simulink model "BANSHEE"  (Simulink 8.1)
settings: Solver=ode1  StartTime=0.0  StopTime=inf  FixedStep=Ts  MaxStep=1e-3  RelTol=1e-3
model workspace (MAT data in the model file):
  op_snapshot1 : opcond.OperatingPoint (value not decoded)
PostLoadFcn:
  | BANSHEE_init;
InitFcn:
  | BANSHEE_init;
values from neighbouring files (symbols this model uses):
  Ts = 100E-6    (= 0.0001)    [BANSHEE_init.m]
undefined symbols (not defined in the file or in its folder): F1, F2, F3, fdesignblkfcn, Feeder1_lib, Feeder2_lib, Feeder3_lib, gcbh, generic_ethernet_cb, Left, relay_housing_lib, SM_UtilityService, SS_F1_RELAY_HOUSING, SS_F2_RELAY_HOUSING, SS_F3_RELAY_HOUSING, SS_Feeder1, SS_Feeder2, SS_Feeder3, type, utility_service_lib, V
libraries: breaker_lib x47, rtio_generic_modbus x43, relay_modbus_lib x42, cables_lib x41, transformer_lib x22, Load_lib x20, artemis x18, powerlib x18, rtio_opalrt_common x15, ssn_lib x15, rtlab x14, simulink x10
(part 1 of 5)
settings Model: ARTEMISmethode_block_infos=$$__separator__$$BANSHEE/ARTEMIS Guide$$__separator__$$  Creator=RE25624  LastModifiedBy=RE25624  BufferReuse=off
settings SolverCC: ZeroCrossAlgorithm=Adaptive
settings DataIOCC: ExternalInput=getinputstruct(op_snapshot1)  InitialState=getstatestruct(op_snapshot1)  LimitDataPoints=off  MaxDataPoints=90060  SignalLoggingSaveFormat=Dataset  SaveOutput=off  SignalLogging=off  DSMLogging=off  SaveTime=off  OutputSaveName=result
settings OptimizationCC: BlockReduction=off  OptimizeBlockIOStorage=off  BufferReuse=off  ExpressionFolding=off  LocalBlockOutputs=off
settings DebuggingCC: MaxConsecutiveZCsMsg=warning  IgnoredZcDiagnostic=none  SolverPrmCheckMsg=none  MultiTaskRateTransMsg=warning  FcnCallInpInsideContextMsg=EnableAllAsWarning  FrameProcessingCompatibilityMsg=error  ModelReferenceExtraNoncontSigs=warning  StrictBusMsg=None
settings ModelReferenceCC: UpdateModelReferenceTargets=IfOutOfDate
settings SFSimCC: SFSimEcho=off
settings GRTTargetCC: CodeReplacementLibrary=C89/C90 (ANSI)

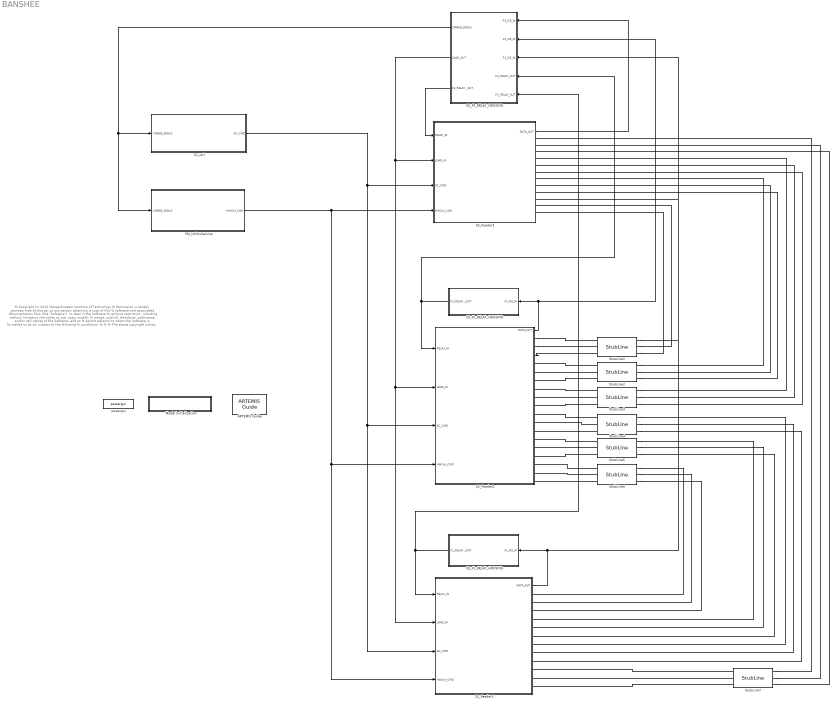
== system BANSHEE ==
  note: % Copyright (c) 2016 Massachusetts Institute of Technology
      | % Permission is hereby granted, free of charge, to any person obtaining a copy of this
      | % software and associated documentation files (the "Software"), to deal in the Software
      | % without restriction, including without limitation the rights to use, copy, modify,
      | % merge, publish, distribute, sublicense, and/or sell copies of the Software, and to
      | % permit persons to whom the Software is furnished to do so, subject to the following
      | % conditions:
      | %
      | %
      | % The above copyright notice and this permission notice shall be included in
      | % all copies or substantial portions of the Software.
      | %
      | % THE SOFTWARE IS PROVIDED "AS IS", WITHOUT WARRANTY OF ANY KIND, EXPRESS OR IMPLIED,
      | % INCLUDING BUT NOT LIMITED TO THE WARRANTIES OF MERCHANTABILITY, FITNESS FOR A
      | % PARTICULAR PURPOSE AND NONINFRINGEMENT. IN NO EVENT SHALL THE AUTHORS OR COPYRIGHT
      | % HOLDERS BE LIABLE FOR ANY CLAIM, DAMAGES OR OTHER LIABILITY, WHETHER IN AN ACTION
      | % OF CONTRACT, TORT OR OTHERWISE, ARISING FROM, OUT OF OR IN CONNECTION WITH THE
      | % SOFTWARE OR THE USE OR OTHER DEALINGS IN THE SOFTWARE.
      | %
      | %
      | %%
  ARTEMIS Guide : artemis/ARTEMIS/ARTEMIS Guide  Tag=FTSSmethode_opal_4hx0r99  Description=5.0_z1  lock=on  Ts=Ts  opt=art5  dyna=off  nb_perm=4  RT_fullcomp=off  ssn=on  ssn_itvc=off  ssn_ivic=off  ssn_ext=off  ssn_solver=Art5 with Backward Euler nodal interface  ssn_impulse=off  ssn_quasimpulse=off  ssn_impulse_loop=5  paraExtinctionThy=off  Thy_Impulse=on  dtc=Off  dtc_opt=normal  ao=on  simtype=off  ct_mac=off  lin_mov=off  lsp=[0.001 2]  spike_skip=Disabled  dtc_extra=1  dtc_sws=normal  dtc_pied=0.5  SPSRulesBlock=SPSRules  tre=on  ctmm=off  LF=off  dpl_type=ARTEMiS DPL  rlc_type=off  custom_type=off  para=on  ssn_ImpulseLoopBlockedStateUpdate=5  ssn_mov_iter_number=5  ssn_switch_iter_number=5
  Model Initialization : Subsystem  AncestorBlock=artemis/Tools /Misc/Model Initialization  mask(Model Functions){InitFcnX=BANSHEE_init;, prel=off, posl=on, inif=on, strf=off}
      mask prompts: InitFcnX "Initialisation"; prel "Preload Function"; posl "PostLoad Function"; inif "InitFcn"; strf "StartFcn"
      mask init:
      | currentBlock = gcb;
      | root = bdroot(currentBlock);
      | 
      | if ~strcmp(get_param(root,'BlockDiagramType'),'library')
      |     if prel==1
      |         set_param(root, 'PreLoadFcn', InitFcnX);
      |     else
      |         set_param(root, 'PreLoadFcn', '');
      |     end
      |     if inif==1
      |         set_param(root, 'InitFcn', InitFcnX);
      |     else
      |         set_param(root, 'InitFcn', '');
      |     end
      |     if strf==1
      |         set_param(root, 'StartFcn', InitFcnX);
      |     else
      |         set_param(root, 'StartFcn', '');
      |     end
      |     if posl==1
      |         set_param(root, 'PostLoadFcn', InitFcnX);
      |     else
      |         set_param(root, 'PostLoadFcn', '');
      |     end
      | end
      | 
      | pos = get_param(currentBlock, 'Position');
      | width = pos(3) - pos(1); height = pos(4) - pos(2);
      | txt = [ upper(root) '\n' '- InitFcn. . . . . '  get_param(root, 'InitFcn') ];
      settings: CopyFcn=set_param(gcb,'LinkStatus','inactive')
      mask Display: text(5, height*0.5, txt, 'horizontalAlignment', 'left', 'verticalAlignment', 'middle') ;
  SC_ctrl : Subsystem
  SM_UtilityService : Subsystem  AncestorBlock=utility_service_lib/SM_UtilityService
  SS_F1_RELAY_HOUSING : Subsystem  AncestorBlock=relay_housing_lib/SS_F1_RELAY_HOUSING
  SS_F2_RELAY_HOUSING : Subsystem  AncestorBlock=relay_housing_lib/SS_F2_RELAY_HOUSING
  SS_F3_RELAY_HOUSING : Subsystem  AncestorBlock=relay_housing_lib/SS_F3_RELAY_HOUSING
  SS_Feeder1 : Subsystem  AncestorBlock=Feeder1_lib/SS_Feeder1
  SS_Feeder2 : Subsystem  AncestorBlock=Feeder2_lib/SS_Feeder2
  SS_Feeder3 : Subsystem  AncestorBlock=Feeder3_lib/SS_Feeder3
  StubLine1 : artemis/ARTEMIS/StubLine  Phases=3  pu=off  L=1500 * 9.43453e-08 / 2  Lpu=0.08  R=1500 * 2.28409e-5 / 2  Rpu=0.002  S_base=450e6/3  V_base=230e3/sqrt(3)  F_base=60  Ts=Ts
  StubLine2 : artemis/ARTEMIS/StubLine  Phases=3  pu=off  L=1500 * 9.43453e-08 / 2  Lpu=0.08  R=1500 * 2.28409e-5 / 2  Rpu=0.002  S_base=450e6/3  V_base=230e3/sqrt(3)  F_base=60  Ts=Ts
  StubLine3 : artemis/ARTEMIS/StubLine  Phases=3  pu=off  L=1500 * 9.43453e-08 / 2  Lpu=0.08  R=1500 * 2.28409e-5 / 2  Rpu=0.002  S_base=450e6/3  V_base=230e3/sqrt(3)  F_base=60  Ts=Ts
  StubLine4 : artemis/ARTEMIS/StubLine  Phases=3  pu=off  L=1000 * 9.43453e-08 / 2  Lpu=0.08  R=1000 * 2.28409e-5 / 2  Rpu=0.002  S_base=450e6/3  V_base=230e3/sqrt(3)  F_base=60  Ts=Ts
  StubLine5 : artemis/ARTEMIS/StubLine  Phases=3  pu=off  L=2000 * 9.43453e-08 / 2  Lpu=0.08  R=2000 * 2.28409e-5 / 2  Rpu=0.002  S_base=450e6/3  V_base=230e3/sqrt(3)  F_base=60  Ts=Ts
  StubLine6 : artemis/ARTEMIS/StubLine  Phases=3  pu=off  L=3000 * 9.43453e-08 / 1  Lpu=0.08  R=3000 * 2.28409e-5 / 1  Rpu=0.002  S_base=450e6/3  V_base=230e3/sqrt(3)  F_base=60  Ts=Ts
  StubLine7 : artemis/ARTEMIS/StubLine  Phases=3  pu=off  L=2000 * 9.43453e-08 / 2  Lpu=0.08  R=2000 * 2.28409e-5 / 2  Rpu=0.002  S_base=450e6/3  V_base=230e3/sqrt(3)  F_base=60  Ts=Ts
  powergui : powerlib/powergui  Priority=2  SimulationMode=Discrete  SolverType=Tustin  SampleTime=Ts  frequency=60  SPID=off  DisableSnubberDevices=off  DisableRonSwitches=off  DisableVfSwitches=off  SwTol=0  Interpol=off  DisplayEquations=off  frequencyindice=0  Pbase=100e6  ErrMax=1e-4  Iterations=50  UnitsV=kV  UnitsW=MW  FunctionMessages=off  echomessages=off  HookPort=off  EnableUseOfTLC=off  x0status=blocks  RestoreLinks=warning  ResistiveCurrentMeasurement=off  Frange=logspace(0,3,50)  Ylog=off  Xlog=off  ShowGrid=off  save=off  variable=ZData  structure=0  ZoomFFT=on  StartTime=0.0  cycles=2  DisplayStyle=off  fundamental=60  FreqAxis=off  MaxFrequency=1000  frequencyindicesteady=1  RmsSteady=1  display=off  Ts=0  methode=off
  wires:
  SS_Feeder3/1(DATA_OUT) -> SS_F3_RELAY_HOUSING/1(F3_MS_IN)
  SS_F3_RELAY_HOUSING/3(F3_RELAY _OUT) -> SS_Feeder3/1(RELAY_IN)
  SS_F1_RELAY_HOUSING/1(F1_RELAY _OUT) -> SS_Feeder1/1(RELAY_IN), SS_F3_RELAY_HOUSING/5(F1_RELAY_OUT)
  SS_F2_RELAY_HOUSING/1(F2_RELAY _OUT) -> SS_F3_RELAY_HOUSING/4(F2_RELAY_OUT), SS_Feeder2/1(RELAY_IN)
  SS_Feeder1/1(DATA_OUT) -> SS_F3_RELAY_HOUSING/3(F1_MS_IN), SS_F1_RELAY_HOUSING/1(F1_MS_IN)
  SS_Feeder2/1(DATA_OUT) -> SS_F3_RELAY_HOUSING/2(F2_MS_IN), SS_F2_RELAY_HOUSING/1(F2_MS_IN)
  SC_ctrl/1(SC_CMD) -> SS_Feeder1/3(SC_CMD), SS_Feeder2/3(SC_CMD), SS_Feeder3/3(SC_CMD)
  SS_F3_RELAY_HOUSING/2(LOAD_OUT) -> SS_Feeder3/2(LOAD_IN), SS_Feeder1/2(LOAD_IN), SS_Feeder2/2(LOAD_IN)
  SM_UtilityService/1(HWCtrl_CMD) -> SS_Feeder1/4(HWCtrl_CMD), SS_Feeder2/4(HWCtrl_CMD), SS_Feeder3/4(HWCtrl_CMD)
  SS_F3_RELAY_HOUSING/1(CMBNE_SGNLS) -> SM_UtilityService/1(CMBNE_SGNLS), SC_ctrl/1(CMBNE_SGNLS)
  connections:
  SS_Feeder2/RConn2 -- StubLine1/LConn2
  SS_Feeder2/RConn1 -- StubLine1/LConn1
  SS_Feeder2/RConn3 -- StubLine1/LConn3
  StubLine2/LConn2 -- SS_Feeder2/RConn5
  StubLine2/LConn3 -- SS_Feeder2/RConn6
  StubLine2/LConn1 -- SS_Feeder2/RConn4
  StubLine3/LConn2 -- SS_Feeder2/RConn8
  StubLine3/LConn1 -- SS_Feeder2/RConn7
  StubLine3/LConn3 -- SS_Feeder2/RConn9
  StubLine4/LConn3 -- SS_Feeder2/RConn12
  StubLine4/LConn2 -- SS_Feeder2/RConn11
  StubLine4/LConn1 -- SS_Feeder2/RConn10
  StubLine7/LConn3 -- SS_Feeder1/RConn12
  StubLine7/LConn2 -- SS_Feeder1/RConn11
  StubLine7/LConn1 -- SS_Feeder1/RConn10
  StubLine5/LConn2 -- SS_Feeder2/RConn14
  StubLine5/LConn1 -- SS_Feeder2/RConn13
  StubLine5/LConn3 -- SS_Feeder2/RConn15
  StubLine6/LConn3 -- SS_Feeder2/RConn18
  StubLine6/LConn2 -- SS_Feeder2/RConn17
  StubLine6/LConn1 -- SS_Feeder2/RConn16
  StubLine6/RConn1 -- SS_Feeder1/RConn1
  StubLine6/RConn2 -- SS_Feeder1/RConn2
  StubLine6/RConn3 -- SS_Feeder1/RConn3
  StubLine5/RConn1 -- SS_Feeder1/RConn4
  StubLine5/RConn2 -- SS_Feeder1/RConn5
  StubLine5/RConn3 -- SS_Feeder1/RConn6
  StubLine4/RConn1 -- SS_Feeder1/RConn7
  StubLine4/RConn2 -- SS_Feeder1/RConn8
  StubLine4/RConn3 -- SS_Feeder1/RConn9
  StubLine3/RConn3 -- SS_Feeder3/RConn6
  StubLine3/RConn2 -- SS_Feeder3/RConn5
  StubLine3/RConn1 -- SS_Feeder3/RConn4
  StubLine2/RConn3 -- SS_Feeder3/RConn9
  StubLine2/RConn2 -- SS_Feeder3/RConn8
  StubLine2/RConn1 -- SS_Feeder3/RConn7
  StubLine1/RConn3 -- SS_Feeder3/RConn12
  StubLine1/RConn2 -- SS_Feeder3/RConn11
  StubLine1/RConn1 -- SS_Feeder3/RConn10
  StubLine7/RConn1 -- SS_Feeder3/RConn1
  StubLine7/RConn2 -- SS_Feeder3/RConn2
  StubLine7/RConn3 -- SS_Feeder3/RConn3

== system BANSHEE/Model Initialization ==

== system BANSHEE/SC_ctrl ==
  note: % Copyright (c) 2016 Massachusetts Institute of Technology
      | % Permission is hereby granted, free of charge, to any person obtaining a copy of this
      | % software and associated documentation files (the "Software"), to deal in the Software
      | % without restriction, including without limitation the rights to use, copy, modify,
      | % merge, publish, distribute, sublicense, and/or sell copies of the Software, and to
      | % permit persons to whom the Software is furnished to do so, subject to the following
      | % conditions:
      | %
      | %
      | % The above copyright notice and this permission notice shall be included in
      | % all copies or substantial portions of the Software.
      | %
      | % THE SOFTWARE IS PROVIDED "AS IS", WITHOUT WARRANTY OF ANY KIND, EXPRESS OR IMPLIED,
      | % INCLUDING BUT NOT LIMITED TO THE WARRANTIES OF MERCHANTABILITY, FITNESS FOR A
      | % PARTICULAR PURPOSE AND NONINFRINGEMENT. IN NO EVENT SHALL THE AUTHORS OR COPYRIGHT
      | % HOLDERS BE LIABLE FOR ANY CLAIM, DAMAGES OR OTHER LIABILITY, WHETHER IN AN ACTION
      | % OF CONTRACT, TORT OR OTHERWISE, ARISING FROM, OUT OF OR IN CONNECTION WITH THE
      | % SOFTWARE OR THE USE OR OTHER DEALINGS IN THE SOFTWARE.
      | %
      | %
      | %%
  note: The 'Overruns' value should remain at 0.
      | The 'Ttotal' value should be equal to the
      | model Fixed-Step size.
  CMBNE_SGNLS : Inport
  Bus Creator : BusCreator  Inputs=2
  Bus Creator1 : BusCreator  Inputs=3
  Bus Selector : BusSelector  OutputSignals=F1_RELAY_OUT,F2_RELAY_OUT,F3_RELAY_OUT
  F1 : Subsystem
  F1 1: connect motor 0: disconnect motor1 : Constant  Value=0
  F2 : Subsystem
  F3 : Subsystem
  F3 1: connect motor 0: disconnect motor : Constant  Value=0
  OpComm : rtlab/OpComm  nbport=1  groupe_acq=1  subsys_rate=0  st=0  Synchronization=on  Interpolation=on  Threshold=1.0  Missed_Data=off  Sim_Time=off  Samples=off  dynSigOut=off  from_console=0  warning_done=off  writeOpCommFile=off  Offset=off
  Woodward : Subsystem
  opElectricFaultSelector : artemis/Tools /POW faults/opElectricFaultSelector  phase_a=on  phase_b=on  phase_c=on  gnd_fault=on  Tacq=1  Tst=[0.1 0 10]  enable_POW=off  angle_POW=[15 0 10]  Tdr="[0.5 0  10]"  fault_location_menu=No fault  T_init=2
  SC_CMD : Outport
  wires:
  CMBNE_SGNLS/1 -> OpComm/1
  opElectricFaultSelector/1 -> [fault_cmd]
  Bus Creator1/1 -> SC_CMD/1
  [IO_ctrl] -> Bus Creator1/3  "IO ctrl"
  Woodward/1(IOctrl) -> [IO_ctrl]
  [fault_cmd] -> Bus Creator1/1  "fault_cmd"
  OpComm/1 -> Bus Selector/1
  Bus Creator/1 -> Bus Creator1/2  "motor_ONOFF"
  F3 1: connect motor 0: disconnect motor/1 -> Bus Creator/1  "F3_motor_ONOFF"
  F1 1: connect motor 0: disconnect motor1/1 -> Bus Creator/2  "F1_motor_ONOFF"
  Bus Selector/1 -> F1/1(F1)  "<F1_RELAY_OUT>"
  Bus Selector/3 -> F3/1(F3)  "<F3_RELAY_OUT>"
  Bus Selector/2 -> F2/1(F2)  "<F2_RELAY_OUT>"

== system BANSHEE/SM_UtilityService ==
  note: % Copyright (c) 2016 Massachusetts Institute of Technology
      | % Permission is hereby granted, free of charge, to any person obtaining a copy of this
      | % software and associated documentation files (the "Software"), to deal in the Software
      | % without restriction, including without limitation the rights to use, copy, modify,
      | % merge, publish, distribute, sublicense, and/or sell copies of the Software, and to
      | % permit persons to whom the Software is furnished to do so, subject to the following
      | % conditions:
      | %
      | %
      | % The above copyright notice and this permission notice shall be included in
      | % all copies or substantial portions of the Software.
      | %
      | % THE SOFTWARE IS PROVIDED "AS IS", WITHOUT WARRANTY OF ANY KIND, EXPRESS OR IMPLIED,
      | % INCLUDING BUT NOT LIMITED TO THE WARRANTIES OF MERCHANTABILITY, FITNESS FOR A
      | % PARTICULAR PURPOSE AND NONINFRINGEMENT. IN NO EVENT SHALL THE AUTHORS OR COPYRIGHT
      | % HOLDERS BE LIABLE FOR ANY CLAIM, DAMAGES OR OTHER LIABILITY, WHETHER IN AN ACTION
      | % OF CONTRACT, TORT OR OTHERWISE, ARISING FROM, OUT OF OR IN CONNECTION WITH THE
      | % SOFTWARE OR THE USE OR OTHER DEALINGS IN THE SOFTWARE.
      | %
      | %
      | %%
  CMBNE_SGNLS : Inport
  2X MCB - Genset_signal_scaling - 3.5MVA : EasyGen3500_GensetSignalScaling_lib/2X MCB - Genset_signal_scaling - 3.5MVA  Vpk_mcb=11268  watt_mcb=3150000  Vpk_gcb=11268  watt_gcb=3150000  rated_rpm=1800  wm_noise_bias=0.02
  Bus Creator4 : BusCreator  Inputs=3
  Bus Selector1 : BusSelector  OutputSignals="F1_MS_IN.DIESEL_DATA.DIESEL_GCB.cb_ms,F1_MS_IN.CB_DATA.F1_PCC,F1_MS_IN.DIESEL_DATA.Gen2_meas.w.w.Rotor speed  wm (pu)"
  Bus Selector2 : BusSelector  OutputSignals=F1_MS_IN.CB_DATA.F1_PCC,F2_MS_IN.CB_DATA.F2_PCC,F3_MS_IN.CB_DATA.F3_PCC
  Bus Selector4 : BusSelector  OutputSignals="F3_MS_IN.NG_CHP_DATA.NG_CHP_GCB.cb_ms,F3_MS_IN.CB_DATA.F3_PCC,F3_MS_IN.NG_CHP_DATA.Gen1_meas.w.w.Rotor speed  wm (pu),F3_MS_IN.CB_DATA.F3_CB_3"
  Genset_signal_scaling - 4MVA : EasyGen3500_GensetSignalScaling_lib/Genset_signal_scaling - 4MVA  Vpk_mcb=11268  watt_mcb=3600000  Vpk_gcb=11268  watt_gcb=3600000  rated_rpm=1800  wm_noise_bias=0.02
  HWCtrl_IOs : Subsystem
  Memory1 : Memory
  OpComm2 : rtlab/OpComm  nbport=1  groupe_acq=1  subsys_rate=0  st=0  Synchronization=on  Interpolation=on  Threshold=1.0  Missed_Data=off  Sim_Time=off  Samples=off  dynSigOut=off  from_console=0  warning_done=off  writeOpCommFile=off  Offset=off
  SEL751 - SignalScaling : Subsystem  mask(SEL751 - SignalScaling){ct_ratio=1/1250, pt_ratio=1/1800}
      mask prompts: ct_ratio "CT Ratio"; pt_ratio "PT Ratio"
      mask help: CT and PT ratios should match the settings in the corresponding SEL751
  HWCtrl_CMD : Outport
  wires:
  Memory1/1 -> HWCtrl_CMD/1
  2X MCB - Genset_signal_scaling - 3.5MVA/1 -> Bus Creator4/1  "NGCHP_ScaledSignals"
  Genset_signal_scaling - 4MVA/1 -> Bus Creator4/2  "Diesel_ScaledSignals"
  [CMBNE_SGNLS] -> Bus Selector4/1, Bus Selector2/1, Bus Selector1/1  "MCB"
  Bus Selector4/3 -> 2X MCB - Genset_signal_scaling - 3.5MVA/3  "<Rotor speed  wm (pu)>"
  Bus Selector4/2 -> 2X MCB - Genset_signal_scaling - 3.5MVA/2  "<F3_PCC>"
  Bus Selector4/1 -> 2X MCB - Genset_signal_scaling - 3.5MVA/1  "<cb_ms>"
  Bus Creator4/1 -> HWCtrl_IOs/1(ScaledSignals)
  HWCtrl_IOs/1(WoodwardBias) -> Memory1/1
  Bus Selector1/3 -> Genset_signal_scaling - 4MVA/3  "<Rotor speed  wm (pu)>"
  Bus Selector1/2 -> Genset_signal_scaling - 4MVA/2  "<F1_PCC>"
  Bus Selector1/1 -> Genset_signal_scaling - 4MVA/1  "<cb_ms>"
  CMBNE_SGNLS/1 -> OpComm2/1
  OpComm2/1 -> [CMBNE_SGNLS]
  SEL751 - SignalScaling/1(ScaledSignals) -> Bus Creator4/3  "SEL751_ScaledSignals"
  Bus Selector2/2 -> SEL751 - SignalScaling/2(Relay_F2)  "<F2_PCC>"
  Bus Selector2/1 -> SEL751 - SignalScaling/1(Relay_F1)  "<F1_PCC>"
  Bus Selector2/3 -> SEL751 - SignalScaling/3(Relay_F3)  "<F3_PCC>"
  Bus Selector4/4 -> 2X MCB - Genset_signal_scaling - 3.5MVA/4  "<F3_CB_3>"

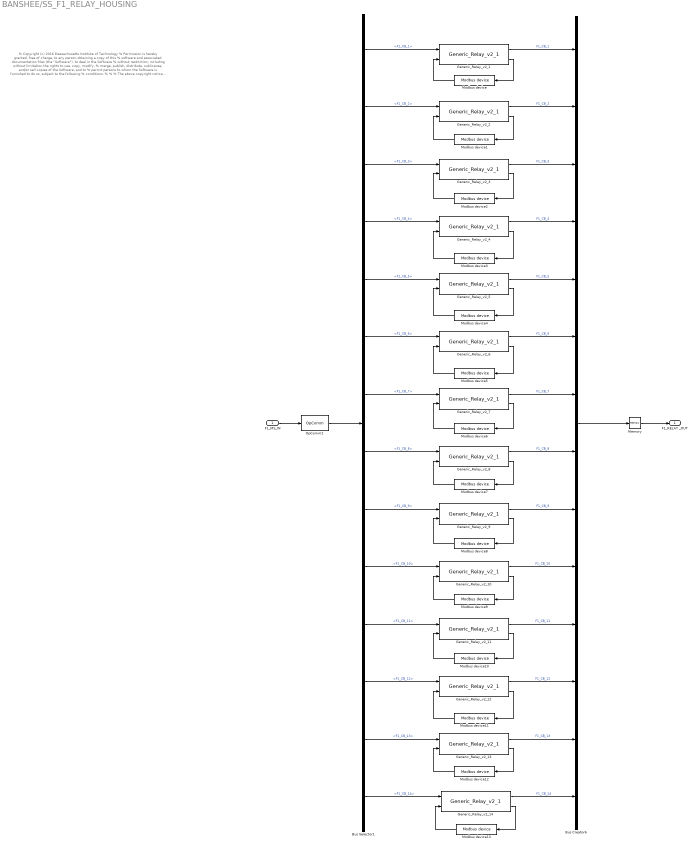
== system BANSHEE/SS_F1_RELAY_HOUSING ==
  note: % Copyright (c) 2016 Massachusetts Institute of Technology
      | % Permission is hereby granted, free of charge, to any person obtaining a copy of this
      | % software and associated documentation files (the "Software"), to deal in the Software
      | % without restriction, including without limitation the rights to use, copy, modify,
      | % merge, publish, distribute, sublicense, and/or sell copies of the Software, and to
      | % permit persons to whom the Software is furnished to do so, subject to the following
      | % conditions:
      | %
      | %
      | % The above copyright notice and this permission notice shall be included in
      | % all copies or substantial portions of the Software.
      | %
      | % THE SOFTWARE IS PROVIDED "AS IS", WITHOUT WARRANTY OF ANY KIND, EXPRESS OR IMPLIED,
      | % INCLUDING BUT NOT LIMITED TO THE WARRANTIES OF MERCHANTABILITY, FITNESS FOR A
      | % PARTICULAR PURPOSE AND NONINFRINGEMENT. IN NO EVENT SHALL THE AUTHORS OR COPYRIGHT
      | % HOLDERS BE LIABLE FOR ANY CLAIM, DAMAGES OR OTHER LIABILITY, WHETHER IN AN ACTION
      | % OF CONTRACT, TORT OR OTHERWISE, ARISING FROM, OUT OF OR IN CONNECTION WITH THE
      | % SOFTWARE OR THE USE OR OTHER DEALINGS IN THE SOFTWARE.
      | %
      | %
      | %%
  F1_MS_IN : Inport
  Bus Creator6 : BusCreator  Inputs=14
  Bus Selector1 : BusSelector  OutputSignals=CB_DATA.F1_CB_1,CB_DATA.F1_CB_2,CB_DATA.F1_CB_3,CB_DATA.F1_CB_4,CB_DATA.F1_CB_5,CB_DATA.F1_CB_6,CB_DATA.F1_CB_7,CB_DATA.F1_CB_8,CB_DATA.F1_CB_9,CB_DATA.F1_CB_10,CB_DATA.F1_CB_11,CB_DATA.F1_CB_12,CB_DATA.F1_CB_13,CB_DATA.F1_CB_14
  Generic_Relay_v2_1 : relay_modbus_lib/Generic_Relay_v2_1  Ts=Ts  relay_settings=[F1(1,:)]
  Generic_Relay_v2_10 : relay_modbus_lib/Generic_Relay_v2_1  Ts=Ts  relay_settings=[F1(10,:)]
  Generic_Relay_v2_11 : relay_modbus_lib/Generic_Relay_v2_1  Ts=Ts  relay_settings=[F1(11,:)]
  Generic_Relay_v2_12 : relay_modbus_lib/Generic_Relay_v2_1  Ts=Ts  relay_settings=[F1(12,:)]
  Generic_Relay_v2_13 : relay_modbus_lib/Generic_Relay_v2_1  Ts=Ts  relay_settings=[F1(13,:)]
  Generic_Relay_v2_14 : relay_modbus_lib/Generic_Relay_v2_1  Ts=Ts  relay_settings=[F1(14,:)]
  Generic_Relay_v2_2 : relay_modbus_lib/Generic_Relay_v2_1  Ts=Ts  relay_settings=[F1(2,:)]
  Generic_Relay_v2_3 : relay_modbus_lib/Generic_Relay_v2_1  Ts=Ts  relay_settings=[F1(3,:)]
  Generic_Relay_v2_4 : relay_modbus_lib/Generic_Relay_v2_1  Ts=Ts  relay_settings=[F1(4,:)]
  Generic_Relay_v2_5 : relay_modbus_lib/Generic_Relay_v2_1  Ts=Ts  relay_settings=[F1(5,:)]
  Generic_Relay_v2_6 : relay_modbus_lib/Generic_Relay_v2_1  Ts=Ts  relay_settings=[F1(6,:)]
  Generic_Relay_v2_7 : relay_modbus_lib/Generic_Relay_v2_1  Ts=Ts  relay_settings=[F1(7,:)]
  Generic_Relay_v2_8 : relay_modbus_lib/Generic_Relay_v2_1  Ts=Ts  relay_settings=[F1(8,:)]
  Generic_Relay_v2_9 : relay_modbus_lib/Generic_Relay_v2_1  Ts=Ts  relay_settings=[F1(9,:)]
  Memory : Memory
  Modbus device : rtio_generic_modbus/Modbus device  conf_name=F1_relay_cfg1.opal  conf_name_mask=F1_relay_cfg1.xls  sample_time=Ts
  Modbus device1 : rtio_generic_modbus/Modbus device  conf_name=F1_relay_cfg2.opal  conf_name_mask=F1_relay_cfg2.xls  sample_time=Ts
  Modbus device10 : rtio_generic_modbus/Modbus device  conf_name=F1_relay_cfg11.opal  conf_name_mask=F1_relay_cfg11.xls  sample_time=Ts
  Modbus device11 : rtio_generic_modbus/Modbus device  conf_name=F1_relay_cfg12.opal  conf_name_mask=F1_relay_cfg12.xls  sample_time=Ts
  Modbus device12 : rtio_generic_modbus/Modbus device  conf_name=F1_relay_cfg13.opal  conf_name_mask=F1_relay_cfg13.xls  sample_time=Ts
  Modbus device13 : rtio_generic_modbus/Modbus device  conf_name=F1_relay_cfg14.opal  conf_name_mask=F1_relay_cfg14.xls  sample_time=Ts
  Modbus device2 : rtio_generic_modbus/Modbus device  conf_name=F1_relay_cfg3.opal  conf_name_mask=F1_relay_cfg3.xls  sample_time=Ts
  Modbus device3 : rtio_generic_modbus/Modbus device  conf_name=F1_relay_cfg4.opal  conf_name_mask=F1_relay_cfg4.xls  sample_time=Ts
  Modbus device4 : rtio_generic_modbus/Modbus device  conf_name=F1_relay_cfg5.opal  conf_name_mask=F1_relay_cfg5.xls  sample_time=Ts
  Modbus device5 : rtio_generic_modbus/Modbus device  conf_name=F1_relay_cfg6.opal  conf_name_mask=F1_relay_cfg6.xls  sample_time=Ts
  Modbus device6 : rtio_generic_modbus/Modbus device  conf_name=F1_relay_cfg7.opal  conf_name_mask=F1_relay_cfg7.xls  sample_time=Ts
  Modbus device7 : rtio_generic_modbus/Modbus device  conf_name=F1_relay_cfg8.opal  conf_name_mask=F1_relay_cfg8.xls  sample_time=Ts
  Modbus device8 : rtio_generic_modbus/Modbus device  conf_name=F1_relay_cfg9.opal  conf_name_mask=F1_relay_cfg9.xls  sample_time=Ts
  Modbus device9 : rtio_generic_modbus/Modbus device  conf_name=F1_relay_cfg10.opal  conf_name_mask=F1_relay_cfg10.xls  sample_time=Ts
  OpComm2 : rtlab/OpComm  nbport=1  groupe_acq=1  subsys_rate=0  st=0  Synchronization=on  Interpolation=on  Threshold=1.0  Missed_Data=off  Sim_Time=off  Samples=off  dynSigOut=off  from_console=0  warning_done=off  writeOpCommFile=off  Offset=off
  F1_RELAY _OUT : Outport
  wires:
  OpComm2/1 -> Bus Selector1/1
  Modbus device12/1 -> Generic_Relay_v2_13/2
  Generic_Relay_v2_13/2 -> Modbus device12/1
  Modbus device11/1 -> Generic_Relay_v2_12/2
  Generic_Relay_v2_12/2 -> Modbus device11/1
  Modbus device10/1 -> Generic_Relay_v2_11/2
  Generic_Relay_v2_11/2 -> Modbus device10/1
  Modbus device9/1 -> Generic_Relay_v2_10/2
  Generic_Relay_v2_10/2 -> Modbus device9/1
  Modbus device8/1 -> Generic_Relay_v2_9/2
  Generic_Relay_v2_9/2 -> Modbus device8/1
  Modbus device7/1 -> Generic_Relay_v2_8/2
  Generic_Relay_v2_8/2 -> Modbus device7/1
  Modbus device6/1 -> Generic_Relay_v2_7/2
  Generic_Relay_v2_7/2 -> Modbus device6/1
  Modbus device5/1 -> Generic_Relay_v2_6/2
  Generic_Relay_v2_6/2 -> Modbus device5/1
  Modbus device4/1 -> Generic_Relay_v2_5/2
  Generic_Relay_v2_5/2 -> Modbus device4/1
  Modbus device3/1 -> Generic_Relay_v2_4/2
  Generic_Relay_v2_4/2 -> Modbus device3/1
  Modbus device2/1 -> Generic_Relay_v2_3/2
  Generic_Relay_v2_3/2 -> Modbus device2/1
  Generic_Relay_v2_2/2 -> Modbus device1/1
  Modbus device1/1 -> Generic_Relay_v2_2/2
  Generic_Relay_v2_1/2 -> Modbus device/1
  Modbus device/1 -> Generic_Relay_v2_1/2
  F1_MS_IN/1 -> OpComm2/1
  Bus Selector1/1 -> Generic_Relay_v2_1/1  "<F1_CB_1>"
  Generic_Relay_v2_1/1 -> Bus Creator6/1  "F1_CB_1"
  Bus Creator6/1 -> Memory/1
  Bus Selector1/2 -> Generic_Relay_v2_2/1  "<F1_CB_2>"
  Generic_Relay_v2_2/1 -> Bus Creator6/2  "F1_CB_2"
  Bus Selector1/3 -> Generic_Relay_v2_3/1  "<F1_CB_3>"
  Bus Selector1/4 -> Generic_Relay_v2_4/1  "<F1_CB_4>"
  Bus Selector1/5 -> Generic_Relay_v2_5/1  "<F1_CB_5>"
  Bus Selector1/6 -> Generic_Relay_v2_6/1  "<F1_CB_6>"
  Bus Selector1/7 -> Generic_Relay_v2_7/1  "<F1_CB_7>"
  Bus Selector1/8 -> Generic_Relay_v2_8/1  "<F1_CB_8>"
  Bus Selector1/9 -> Generic_Relay_v2_9/1  "<F1_CB_9>"
  Bus Selector1/10 -> Generic_Relay_v2_10/1  "<F1_CB_10>"
  Bus Selector1/11 -> Generic_Relay_v2_11/1  "<F1_CB_11>"
  Bus Selector1/12 -> Generic_Relay_v2_12/1  "<F1_CB_12>"
  Bus Selector1/13 -> Generic_Relay_v2_13/1  "<F1_CB_13>"
  Generic_Relay_v2_13/1 -> Bus Creator6/13  "F1_CB_13"
  Generic_Relay_v2_12/1 -> Bus Creator6/12  "F1_CB_12"
  Generic_Relay_v2_11/1 -> Bus Creator6/11  "F1_CB_11"
  Generic_Relay_v2_10/1 -> Bus Creator6/10  "F1_CB_10"
  Generic_Relay_v2_9/1 -> Bus Creator6/9  "F1_CB_9"
  Generic_Relay_v2_8/1 -> Bus Creator6/8  "F1_CB_8"
  Generic_Relay_v2_7/1 -> Bus Creator6/7  "F1_CB_7"
  Generic_Relay_v2_6/1 -> Bus Creator6/6  "F1_CB_6"
  Generic_Relay_v2_5/1 -> Bus Creator6/5  "F1_CB_5"
  Generic_Relay_v2_4/1 -> Bus Creator6/4  "F1_CB_4"
  Generic_Relay_v2_3/1 -> Bus Creator6/3  "F1_CB_3"
  Modbus device13/1 -> Generic_Relay_v2_14/2
  Generic_Relay_v2_14/2 -> Modbus device13/1
  Generic_Relay_v2_14/1 -> Bus Creator6/14  "F1_CB_14"
  Bus Selector1/14 -> Generic_Relay_v2_14/1  "<F1_CB_14>"
  Memory/1 -> F1_RELAY _OUT/1

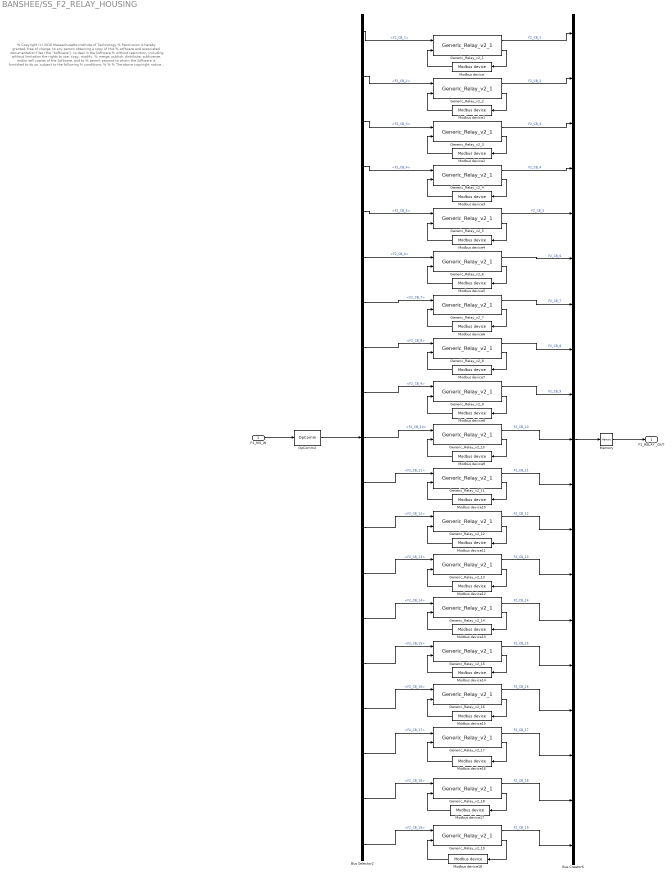
== system BANSHEE/SS_F2_RELAY_HOUSING ==
  note: % Copyright (c) 2016 Massachusetts Institute of Technology
      | % Permission is hereby granted, free of charge, to any person obtaining a copy of this
      | % software and associated documentation files (the "Software"), to deal in the Software
      | % without restriction, including without limitation the rights to use, copy, modify,
      | % merge, publish, distribute, sublicense, and/or sell copies of the Software, and to
      | % permit persons to whom the Software is furnished to do so, subject to the following
      | % conditions:
      | %
      | %
      | % The above copyright notice and this permission notice shall be included in
      | % all copies or substantial portions of the Software.
      | %
      | % THE SOFTWARE IS PROVIDED "AS IS", WITHOUT WARRANTY OF ANY KIND, EXPRESS OR IMPLIED,
      | % INCLUDING BUT NOT LIMITED TO THE WARRANTIES OF MERCHANTABILITY, FITNESS FOR A
      | % PARTICULAR PURPOSE AND NONINFRINGEMENT. IN NO EVENT SHALL THE AUTHORS OR COPYRIGHT
      | % HOLDERS BE LIABLE FOR ANY CLAIM, DAMAGES OR OTHER LIABILITY, WHETHER IN AN ACTION
      | % OF CONTRACT, TORT OR OTHERWISE, ARISING FROM, OUT OF OR IN CONNECTION WITH THE
      | % SOFTWARE OR THE USE OR OTHER DEALINGS IN THE SOFTWARE.
      | %
      | %
      | %%
  F2_MS_IN : Inport
  Bus Creator6 : BusCreator  Inputs=19
  Bus Selector2 : BusSelector  OutputSignals=CB_DATA.F2_CB_1,CB_DATA.F2_CB_2,CB_DATA.F2_CB_3,CB_DATA.F2_CB_4,CB_DATA.F2_CB_5,CB_DATA.F2_CB_6,CB_DATA.F2_CB_7,CB_DATA.F2_CB_8,CB_DATA.F2_CB_9,CB_DATA.F2_CB_10,CB_DATA.F2_CB_11,CB_DATA.F2_CB_12,CB_DATA.F2_CB_13,CB_DATA.F2_CB_14,CB_DATA.F2_CB_15,CB_DATA.F2_CB_16,CB_DATA.F2_CB_17,CB_DATA.F2_CB_18,CB_DATA.F2_CB_19
  Generic_Relay_v2_1 : relay_modbus_lib/Generic_Relay_v2_1  Ts=Ts  relay_settings=[F2(1,:)]
  Generic_Relay_v2_10 : relay_modbus_lib/Generic_Relay_v2_1  Ts=Ts  relay_settings=[F2(10,:)]
  Generic_Relay_v2_11 : relay_modbus_lib/Generic_Relay_v2_1  Ts=Ts  relay_settings=[F2(11,:)]
  Generic_Relay_v2_12 : relay_modbus_lib/Generic_Relay_v2_1  Ts=Ts  relay_settings=[F2(12,:)]
  Generic_Relay_v2_13 : relay_modbus_lib/Generic_Relay_v2_1  Ts=Ts  relay_settings=[F2(13,:)]
  Generic_Relay_v2_14 : relay_modbus_lib/Generic_Relay_v2_1  Ts=Ts  relay_settings=[F2(14,:)]
  Generic_Relay_v2_15 : relay_modbus_lib/Generic_Relay_v2_1  Ts=Ts  relay_settings=[F2(15,:)]
  Generic_Relay_v2_16 : relay_modbus_lib/Generic_Relay_v2_1  Ts=Ts  relay_settings=[F2(16,:)]
  Generic_Relay_v2_17 : relay_modbus_lib/Generic_Relay_v2_1  Ts=Ts  relay_settings=[F2(17,:)]
  Generic_Relay_v2_18 : relay_modbus_lib/Generic_Relay_v2_1  Ts=Ts  relay_settings=[F2(18,:)]
  Generic_Relay_v2_19 : relay_modbus_lib/Generic_Relay_v2_1  Ts=Ts  relay_settings=[F2(19,:)]
  Generic_Relay_v2_2 : relay_modbus_lib/Generic_Relay_v2_1  Ts=Ts  relay_settings=[F2(2,:)]
  Generic_Relay_v2_3 : relay_modbus_lib/Generic_Relay_v2_1  Ts=Ts  relay_settings=[F2(3,:)]
  Generic_Relay_v2_4 : relay_modbus_lib/Generic_Relay_v2_1  Ts=Ts  relay_settings=[F2(4,:)]
  Generic_Relay_v2_5 : relay_modbus_lib/Generic_Relay_v2_1  Ts=Ts  relay_settings=[F2(5,:)]
  Generic_Relay_v2_6 : relay_modbus_lib/Generic_Relay_v2_1  Ts=Ts  relay_settings=[F2(6,:)]
  Generic_Relay_v2_7 : relay_modbus_lib/Generic_Relay_v2_1  Ts=Ts  relay_settings=[F2(7,:)]
  Generic_Relay_v2_8 : relay_modbus_lib/Generic_Relay_v2_1  Ts=Ts  relay_settings=[F2(8,:)]
  Generic_Relay_v2_9 : relay_modbus_lib/Generic_Relay_v2_1  Ts=Ts  relay_settings=[F2(9,:)]
  Memory : Memory
  Modbus device : rtio_generic_modbus/Modbus device  conf_name=F2_relay_cfg1.opal  conf_name_mask=F2_relay_cfg1.xls  sample_time=Ts
  Modbus device1 : rtio_generic_modbus/Modbus device  conf_name=F2_relay_cfg2.opal  conf_name_mask=F2_relay_cfg2.xls  sample_time=Ts
  Modbus device10 : rtio_generic_modbus/Modbus device  conf_name=F2_relay_cfg11.opal  conf_name_mask=F2_relay_cfg11.xls  sample_time=Ts
  Modbus device11 : rtio_generic_modbus/Modbus device  conf_name=F2_relay_cfg12.opal  conf_name_mask=F2_relay_cfg12.xls  sample_time=Ts
  Modbus device12 : rtio_generic_modbus/Modbus device  conf_name=F2_relay_cfg13.opal  conf_name_mask=F2_relay_cfg13.xls  sample_time=Ts
  Modbus device13 : rtio_generic_modbus/Modbus device  conf_name=F2_relay_cfg14.opal  conf_name_mask=F2_relay_cfg14.xls  sample_time=Ts
  Modbus device14 : rtio_generic_modbus/Modbus device  conf_name=F2_relay_cfg15.opal  conf_name_mask=F2_relay_cfg15.xls  sample_time=Ts
  Modbus device15 : rtio_generic_modbus/Modbus device  conf_name=F2_relay_cfg16.opal  conf_name_mask=F2_relay_cfg16.xls  sample_time=Ts
  Modbus device16 : rtio_generic_modbus/Modbus device  conf_name=F2_relay_cfg17.opal  conf_name_mask=F2_relay_cfg17.xls  sample_time=Ts
  Modbus device17 : rtio_generic_modbus/Modbus device  conf_name=F2_relay_cfg18.opal  conf_name_mask=F2_relay_cfg18.xls  sample_time=Ts
  Modbus device18 : rtio_generic_modbus/Modbus device  conf_name=F2_relay_cfg19.opal  conf_name_mask=F2_relay_cfg19.xls  sample_time=Ts
  Modbus device2 : rtio_generic_modbus/Modbus device  conf_name=F2_relay_cfg3.opal  conf_name_mask=F2_relay_cfg3.xls  sample_time=Ts
  Modbus device3 : rtio_generic_modbus/Modbus device  conf_name=F2_relay_cfg4.opal  conf_name_mask=F2_relay_cfg4.xls  sample_time=Ts
  Modbus device4 : rtio_generic_modbus/Modbus device  conf_name=F2_relay_cfg5.opal  conf_name_mask=F2_relay_cfg5.xls  sample_time=Ts
  Modbus device5 : rtio_generic_modbus/Modbus device  conf_name=F2_relay_cfg6.opal  conf_name_mask=F2_relay_cfg6.xls  sample_time=Ts
  Modbus device6 : rtio_generic_modbus/Modbus device  conf_name=F2_relay_cfg7.opal  conf_name_mask=F2_relay_cfg7.xls  sample_time=Ts
  Modbus device7 : rtio_generic_modbus/Modbus device  conf_name=F2_relay_cfg8.opal  conf_name_mask=F2_relay_cfg8.xls  sample_time=Ts
  Modbus device8 : rtio_generic_modbus/Modbus device  conf_name=F2_relay_cfg9.opal  conf_name_mask=F2_relay_cfg9.xls  sample_time=Ts
  Modbus device9 : rtio_generic_modbus/Modbus device  conf_name=F2_relay_cfg10.opal  conf_name_mask=F2_relay_cfg10.xls  sample_time=Ts
  OpComm2 : rtlab/OpComm  nbport=1  groupe_acq=1  subsys_rate=0  st=0  Synchronization=on  Interpolation=on  Threshold=1.0  Missed_Data=off  Sim_Time=off  Samples=off  dynSigOut=off  from_console=0  warning_done=off  writeOpCommFile=off  Offset=off
  F2_RELAY _OUT : Outport
  wires:
  OpComm2/1 -> Bus Selector2/1
  Modbus device16/1 -> Generic_Relay_v2_17/2
  Generic_Relay_v2_17/2 -> Modbus device16/1
  Modbus device15/1 -> Generic_Relay_v2_16/2
  Generic_Relay_v2_16/2 -> Modbus device15/1
  Modbus device14/1 -> Generic_Relay_v2_15/2
  Generic_Relay_v2_15/2 -> Modbus device14/1
  Modbus device13/1 -> Generic_Relay_v2_14/2
  Generic_Relay_v2_14/2 -> Modbus device13/1
  Generic_Relay_v2_13/2 -> Modbus device12/1
  Modbus device12/1 -> Generic_Relay_v2_13/2
  Modbus device11/1 -> Generic_Relay_v2_12/2
  Generic_Relay_v2_12/2 -> Modbus device11/1
  Modbus device10/1 -> Generic_Relay_v2_11/2
  Generic_Relay_v2_11/2 -> Modbus device10/1
  Modbus device9/1 -> Generic_Relay_v2_10/2
  Generic_Relay_v2_10/2 -> Modbus device9/1
  Modbus device8/1 -> Generic_Relay_v2_9/2
  Generic_Relay_v2_9/2 -> Modbus device8/1
  Modbus device7/1 -> Generic_Relay_v2_8/2
  Generic_Relay_v2_8/2 -> Modbus device7/1
  Modbus device6/1 -> Generic_Relay_v2_7/2
  Generic_Relay_v2_7/2 -> Modbus device6/1
  Generic_Relay_v2_6/2 -> Modbus device5/1
  Modbus device5/1 -> Generic_Relay_v2_6/2
  Modbus device4/1 -> Generic_Relay_v2_5/2
  Generic_Relay_v2_5/2 -> Modbus device4/1
  Modbus device3/1 -> Generic_Relay_v2_4/2
  Generic_Relay_v2_4/2 -> Modbus device3/1
  Modbus device2/1 -> Generic_Relay_v2_3/2
  Generic_Relay_v2_3/2 -> Modbus device2/1
  Modbus device1/1 -> Generic_Relay_v2_2/2
  Generic_Relay_v2_2/2 -> Modbus device1/1
  Modbus device/1 -> Generic_Relay_v2_1/2
  Generic_Relay_v2_1/2 -> Modbus device/1
  Bus Creator6/1 -> Memory/1
  F2_MS_IN/1 -> OpComm2/1
  Bus Selector2/1 -> Generic_Relay_v2_1/1  "<F2_CB_1>"
  Generic_Relay_v2_1/1 -> Bus Creator6/1  "F2_CB_1"
  Bus Selector2/2 -> Generic_Relay_v2_2/1  "<F2_CB_2>"
  Bus Selector2/3 -> Generic_Relay_v2_3/1  "<F2_CB_3>"
  Bus Selector2/4 -> Generic_Relay_v2_4/1  "<F2_CB_4>"
  Bus Selector2/5 -> Generic_Relay_v2_5/1  "<F2_CB_5>"
  Bus Selector2/6 -> Generic_Relay_v2_6/1  "<F2_CB_6>"
  Bus Selector2/7 -> Generic_Relay_v2_7/1  "<F2_CB_7>"
  Bus Selector2/8 -> Generic_Relay_v2_8/1  "<F2_CB_8>"
  Bus Selector2/9 -> Generic_Relay_v2_9/1  "<F2_CB_9>"
  Bus Selector2/10 -> Generic_Relay_v2_10/1  "<F2_CB_10>"
  Bus Selector2/11 -> Generic_Relay_v2_11/1  "<F2_CB_11>"
  Bus Selector2/12 -> Generic_Relay_v2_12/1  "<F2_CB_12>"
  Bus Selector2/13 -> Generic_Relay_v2_13/1  "<F2_CB_13>"
  Bus Selector2/14 -> Generic_Relay_v2_14/1  "<F2_CB_14>"
  Bus Selector2/15 -> Generic_Relay_v2_15/1  "<F2_CB_15>"
  Bus Selector2/16 -> Generic_Relay_v2_16/1  "<F2_CB_16>"
  Generic_Relay_v2_12/1 -> Bus Creator6/12  "F2_CB_12"
  Generic_Relay_v2_13/1 -> Bus Creator6/13  "F2_CB_13"
  Generic_Relay_v2_14/1 -> Bus Creator6/14  "F2_CB_14"
  Generic_Relay_v2_15/1 -> Bus Creator6/15  "F2_CB_15"
  Generic_Relay_v2_16/1 -> Bus Creator6/16  "F2_CB_16"
  Generic_Relay_v2_11/1 -> Bus Creator6/11  "F2_CB_11"
  Generic_Relay_v2_10/1 -> Bus Creator6/10  "F2_CB_10"
  Generic_Relay_v2_9/1 -> Bus Creator6/9  "F2_CB_9"
  Generic_Relay_v2_8/1 -> Bus Creator6/8  "F2_CB_8"
  Generic_Relay_v2_7/1 -> Bus Creator6/7  "F2_CB_7"
  Generic_Relay_v2_2/1 -> Bus Creator6/2  "F2_CB_2"
  Generic_Relay_v2_3/1 -> Bus Creator6/3  "F2_CB_3"
  Generic_Relay_v2_4/1 -> Bus Creator6/4  "F2_CB_4"
  Generic_Relay_v2_5/1 -> Bus Creator6/5  "F2_CB_5"
  Generic_Relay_v2_6/1 -> Bus Creator6/6  "F2_CB_6"
  Generic_Relay_v2_17/1 -> Bus Creator6/17  "F2_CB_17"
  Bus Selector2/17 -> Generic_Relay_v2_17/1  "<F2_CB_17>"
  Modbus device18/1 -> Generic_Relay_v2_19/2
  Generic_Relay_v2_19/2 -> Modbus device18/1
  Modbus device17/1 -> Generic_Relay_v2_18/2
  Generic_Relay_v2_18/2 -> Modbus device17/1
  Generic_Relay_v2_18/1 -> Bus Creator6/18  "F2_CB_18"
  Generic_Relay_v2_19/1 -> Bus Creator6/19  "F2_CB_19"
  Bus Selector2/19 -> Generic_Relay_v2_19/1  "<F2_CB_19>"
  Bus Selector2/18 -> Generic_Relay_v2_18/1  "<F2_CB_18>"
  Memory/1 -> F2_RELAY _OUT/1
